simulink model "steuerung_mdl"  (R2013b)
settings: Solver=ode45  StartTime=0.0  StopTime=0.5  RelTol=1e-3
values from neighbouring files (symbols this model uses):
  K = 0.05    [steuerung.m]
  Kg = K / (K*K + a*R)    (= 16.6666666667)    [steuerung.m]
  Kg_s = 0.9*Kg    (= 15)    [steuerung.m]
  mmax = 0    [steuerung.m]
  R = 0.5    [steuerung.m]
  tau = J*R / (K*K + a*R)    (= 0.0416666666667)    [steuerung.m]
settings Model: Creator=daniw  LastModifiedBy=daniw

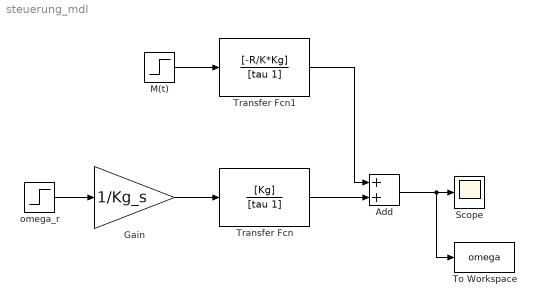
== system steuerung_mdl ==
  Add : Sum
  Gain : Gain  Gain=1/Kg_s
  M(t) : Step  Time=0.3  After=mmax  SampleTime=0
  Scope : Scope
  To Workspace : ToWorkspace  VariableName=omega  SampleTime=-1  SaveFormat=Structure With Time
  Transfer Fcn : TransferFcn  Numerator=[Kg]  Denominator=[tau 1]
  Transfer Fcn1 : TransferFcn  Numerator=[-R/K*Kg]  Denominator=[tau 1]
  omega_r : Step  Time=0.1  Before=5  After=20  SampleTime=0
  wires:
  M(t)/1 -> Transfer Fcn1/1
  omega_r/1 -> Gain/1
  Add/1 -> To Workspace/1, Scope/1
  Transfer Fcn/1 -> Add/2
  Transfer Fcn1/1 -> Add/1
  Gain/1 -> Transfer Fcn/1
